simulink subsystem "subsystem1_trainingMatlab2"  (R2019b)
settings: Solver=VariableStepAuto  StartTime=0.0  StopTime=10.0  RelTol=1e-3
undefined symbols (not defined in the file or in its folder): DiscIntNeverNeededParam
libraries: simulink x1
settings Model: Creator=Laura  LastModifiedBy=Laura

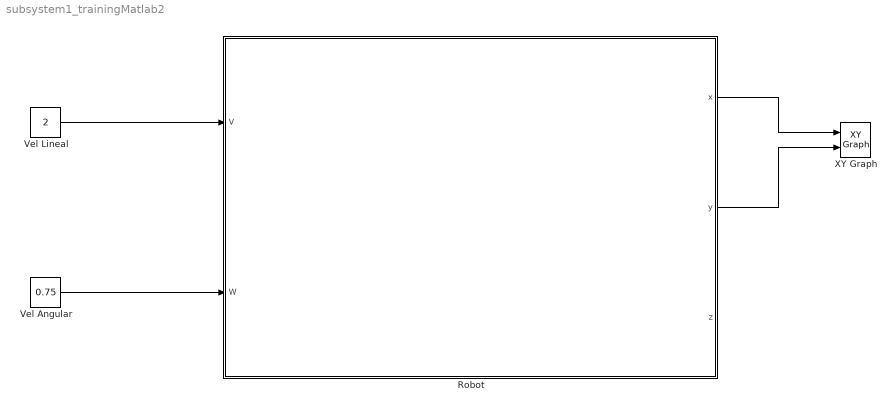
== system subsystem1_trainingMatlab2 ==
  "Robot " : Subsystem
  "Vel Angular " : Constant  Value=0.75
  Vel Lineal : Constant  Value=2
  XY Graph : simulink/Sinks/XY Graph  xmin=-1  xmax=1  ymin=-1  ymax=1  st=-1
  wires:
  "Vel Angular "/1 -> "Robot "/2("W ")
  Vel Lineal/1 -> "Robot "/1("V ")
  "Robot "/2(y) -> XY Graph/2
  "Robot "/1(x) -> XY Graph/1

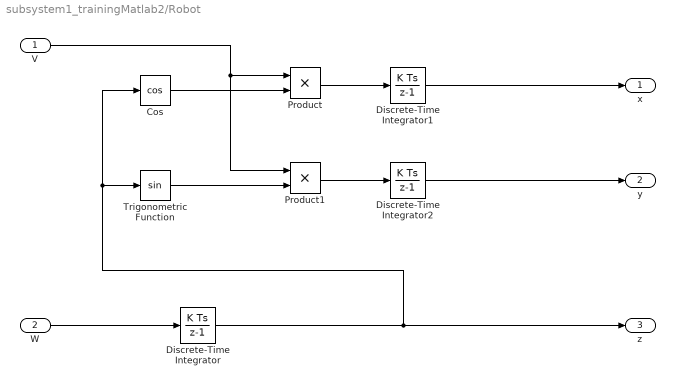
== system subsystem1_trainingMatlab2/Robot  ==
  "V " : Inport
  "W " : Inport  Port=2
  Cos : Trigonometry  Operator=cos
  Discrete-Time Integrator : DiscreteIntegrator  SampleTime=-1  ICPrevOutput=DiscIntNeverNeededParam  ICPrevScaledInput=DiscIntNeverNeededParam
  Discrete-Time Integrator1 : DiscreteIntegrator  SampleTime=-1  ICPrevOutput=DiscIntNeverNeededParam  ICPrevScaledInput=DiscIntNeverNeededParam
  Discrete-Time Integrator2 : DiscreteIntegrator  SampleTime=-1  ICPrevOutput=DiscIntNeverNeededParam  ICPrevScaledInput=DiscIntNeverNeededParam
  Product : Product
  Product1 : Product
  Trigonometric Function : Trigonometry
  x : Outport
  y : Outport  Port=2
  z : Outport  Port=3
  wires:
  Product/1 -> Discrete-Time Integrator1/1
  Trigonometric Function/1 -> Product1/2
  Discrete-Time Integrator/1 -> Cos/1, Trigonometric Function/1, z/1
  "W "/1 -> Discrete-Time Integrator/1
  Discrete-Time Integrator1/1 -> x/1
  Discrete-Time Integrator2/1 -> y/1
  Product1/1 -> Discrete-Time Integrator2/1
  Cos/1 -> Product/2
  "V "/1 -> Product1/1, Product/1
